simulink model "discrM"  (R2018b)
settings: Solver=FixedStepAuto  StartTime=0.0  StopTime=1.0  FixedStep=0.2  RelTol=1e-3  EnableMultiTasking=on
settings Model: Creator=Reichl  LastModifiedBy=Reichl
settings DataIOCC: FinalStateName=xFinalDisc  SaveFinalState=on  SaveCompleteFinalSimState=on  SaveFormat=Array  SaveState=on  StreamToWorkspace=on  SaveTime=off  StateSaveName=xDiscStates
settings OptimizationCC: LifeSpan=inf
settings DebuggingCC: AllowSymbolicDim=off  SFUnexpectedBacktrackingDiag=warning  SFNoUnconditionalDefaultTransitionDiag=warning  SFExecutionAtInitializationDiag=none
settings ModelReferenceCC: PropagateSignalLabelsOutOfModel=off
settings SFSimCC: SimUseLocalCustomCode=off
settings RTWCC: RTWUseLocalCustomCode=off
settings CodeAppCC: StateflowObjectComments=on
settings GRTTargetCC: TargetLangStandard=C89/C90 (ANSI)
settings ConfigComp: CovMetricSettings=dw  CovHtmlReporting=on  CovSaveCumulativeToWorkspaceVar=on  CovSaveSingleToWorkspaceVar=on  CovExternalEMLEnable=off

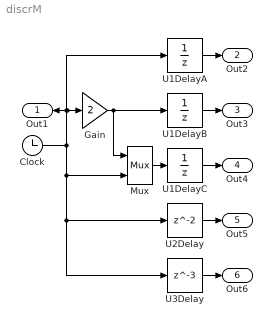
== system discrM ==
  Clock : Clock
  Gain : Gain  Gain=2
  Mux : Mux  Inputs=2
  U1DelayA : UnitDelay  InitialCondition=-2  SampleTime=-1  StateName=DS
  U1DelayB : UnitDelay  InitialCondition=-3  SampleTime=-1  StateName=DS1
  U1DelayC : UnitDelay  InitialCondition=[-40, -41]  SampleTime=-1  StateName=DS2
  U2Delay : Delay  InitialCondition=[-51,-50]  StateName=xd2
  U3Delay : Delay  DelayLength=3  InitialCondition=[-102, -101, -100]  StateName=xd3
  Out1 : Outport
  Out2 : Outport  Port=2
  Out3 : Outport  Port=3
  Out4 : Outport  Port=4
  Out5 : Outport  Port=5
  Out6 : Outport  Port=6
  wires:
  U1DelayA/1 -> Out2/1
  U1DelayB/1 -> Out3/1
  U1DelayC/1 -> Out4/1
  Gain/1 -> U1DelayB/1, Mux/1
  Mux/1 -> U1DelayC/1
  Clock/1 -> Out1/1, Gain/1, U1DelayA/1, U3Delay/1, U2Delay/1, Mux/2
  U2Delay/1 -> Out5/1
  U3Delay/1 -> Out6/1
